simulink model "l3"  (R2013a)
settings: Solver=ode45  StartTime=0.0  StopTime=30  RelTol=1e-3
settings Model: Creator=Sion  LastModifiedBy=Sion

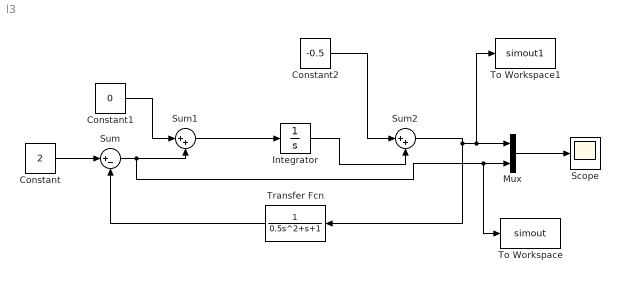
== system l3 ==
  Constant : Constant  Value=2
  Constant1 : Constant  Value=0
  Constant2 : Constant  Value=-0.5
  Integrator : Integrator
  Mux : Mux  Inputs=2
  Scope : Scope
      settings: SaveName=ScopeData18
  Sum : Sum  Inputs=|+-
  Sum1 : Sum  Inputs=|++
  Sum2 : Sum  Inputs=|++
  To Workspace : ToWorkspace  VariableName=simout  SampleTime=-1  SaveFormat=Timeseries
  To Workspace1 : ToWorkspace  VariableName=simout1  SampleTime=-1  SaveFormat=Timeseries
  Transfer Fcn : TransferFcn  Denominator=[0.5 1 1]
  wires:
  Mux/1 -> Scope/1
  Sum1/1 -> Integrator/1
  Constant/1 -> Sum/1
  Sum/1 -> To Workspace/1, Mux/2, Sum1/2
  Constant1/1 -> Sum1/1
  Transfer Fcn/1 -> Sum/2
  Integrator/1 -> Sum2/2
  Constant2/1 -> Sum2/1
  Sum2/1 -> Transfer Fcn/1, To Workspace1/1, Mux/1
